simulink model "Final_3_12_2021"  (R2016a)
settings: Solver=VariableStepAuto  StartTime=0.0  StopTime=10.0  RelTol=1e-3
values from neighbouring files (symbols this model uses):
  A1 = -A(1,1)    [FInal2019.m]    (also in FInal_3_12_2021.m; Final2017.m; Final2018.m; Final2020feb.m)
  A2 = -A(1,2)    [FInal2019.m]    (also in FInal_3_12_2021.m; Final2017.m; Final2018.m; Final2020feb.m)
  K1 = K(1,1)    [FInal2019.m]    (also in FInal_3_12_2021.m = khat(1,1); Final2017.m; Final2018.m; Final2020feb.m = khat(1,1))
  K2 = K(1,2)    [FInal2019.m]    (also in FInal_3_12_2021.m = khat(1,2); Final2017.m; Final2018.m; Final2020feb.m = khat(1,2))
  K3 = K(1,3)    [FInal2019.m]    (also in FInal_3_12_2021.m = khat(1,3); Final2017.m; Final2018.m; Final2020feb.m = khat(1,3))
  Ki = -khat(1,4)    [FInal_3_12_2021.m]    (also in Final2020feb.m)
libraries: simulink x1
settings Model: Creator=alber  LastModifiedBy=alber

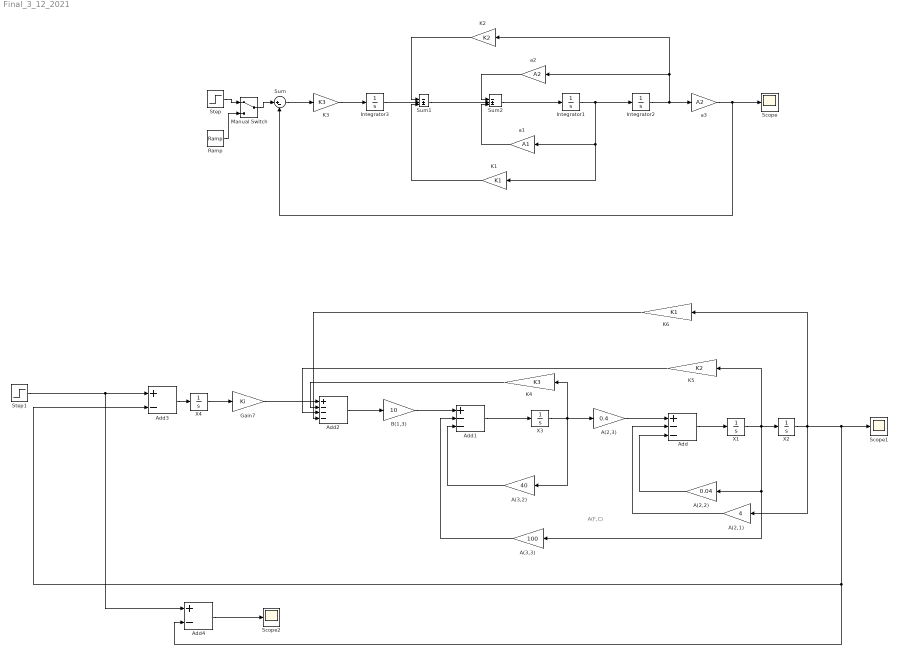
== system Final_3_12_2021 ==
  note: A(F,C)
  A(2,1) : Gain  Gain=4
  A(2,2) : Gain  Gain=0.04
  A(2,3) : Gain  Gain=0.4
  A(3,2) : Gain  Gain=40
  A(3,3) : Gain  Gain=100
  Add : Sum  Inputs=+--
  Add1 : Sum  Inputs=+--
  Add2 : Sum  Inputs=+---
  Add3 : Sum  Inputs=+-
  Add4 : Sum  Inputs=+-
  B(1,3) : Gain  Gain=10
  Gain7 : Gain  Gain=Ki
  Integrator1 : Integrator
  Integrator2 : Integrator
  Integrator3 : Integrator
  K1 : Gain  Gain=K1
  K2 : Gain  Gain=K2
  K3 : Gain  Gain=K3
  K4 : Gain  Gain=K3
  K5 : Gain  Gain=K2
  K6 : Gain  Gain=K1
  Manual Switch : ManualSwitch
  Ramp : simulink/Sources/Ramp  slope=1  start=0  X0=0
  Scope : Scope
  Scope1 : Scope
  Scope2 : Scope
  Step : Step  SampleTime=0
  Step1 : Step  SampleTime=0
  Sum : Sum  Inputs=|+-
  Sum1 : Sum  Inputs=|-+-
  Sum2 : Sum  Inputs=|-+-
  X{1..4} (4 alike) : Integrator
  a1 : Gain  Gain=A1
  a2 : Gain  Gain=A2
  a3 : Gain  Gain=A2
  wires:
  Sum/1 -> K3/1
  K3/1 -> Integrator3/1
  Sum1/1 -> Sum2/2
  Sum2/1 -> Integrator1/1
  Integrator1/1 -> K1/1, a1/1, Integrator2/1
  a1/1 -> Sum2/3
  K1/1 -> Sum1/3
  a2/1 -> Sum2/1
  K2/1 -> Sum1/1
  Integrator2/1 -> a3/1, K2/1, a2/1
  Integrator3/1 -> Sum1/2
  a3/1 -> Scope/1, Sum/2
  Manual Switch/1 -> Sum/1
  Step/1 -> Manual Switch/1
  Ramp/1 -> Manual Switch/2
  X1/1 -> K5/1, A(2,2)/1, A(3,3)/1, X2/1
  Add/1 -> X1/1
  X2/1 -> K6/1, Add4/2, Add3/2, Scope1/1, A(2,1)/1
  A(2,2)/1 -> Add/3
  A(2,1)/1 -> Add/2
  A(2,3)/1 -> Add/1
  X3/1 -> K4/1, A(3,2)/1, A(2,3)/1
  Add1/1 -> X3/1
  A(3,2)/1 -> Add1/3
  A(3,3)/1 -> Add1/2
  B(1,3)/1 -> Add1/1
  Add2/1 -> B(1,3)/1
  K4/1 -> Add2/2
  K5/1 -> Add2/3
  K6/1 -> Add2/4
  Gain7/1 -> Add2/1
  X4/1 -> Gain7/1
  Add3/1 -> X4/1
  Step1/1 -> Add4/1, Add3/1
  Add4/1 -> Scope2/1
